simulink model "sdruFMMonoFPGA"  (R2014a)
settings: Solver=FixedStepDiscrete  SolverMode=SingleTasking  StartTime=0.0  StopTime=inf  RelTol=1e-3
PreLoadFcn:
  | monoFM = getParamsSdruFMMonoDemo;
  | tb = (atan([1, 1/2, 1/4, 1/8, 1/16, 1/32, 1/64, 1/128]));
InitFcn:
  | monoFM = getParamsSdruFMMonoDemo;
  | tb = (atan([1, 1/2, 1/4, 1/8, 1/16, 1/32, 1/64, 1/128]));
undefined symbols (not defined in the file or in its folder): mfilt
libraries: simulink x5, dspmlti4 x1, dsparch4 x1, dspsnks4 x1, sdrublksprivate x1, commsdrhw_v2 x1
CloseFcn:
  | clear monoFM;
  | clear tb
Description:
  | This model uses Universal Software Radio Peripheral (USRP) hardware with Simulink(R) to perform FM mono demodulation.
settings Model: SimulationMode=accelerator  Creator=The MathWorks Inc.
settings DataIOCC: SignalLoggingSaveFormat=ModelDataLogs  SaveOutput=off  SignalLogging=off  DSMLogging=off  SaveTime=off
settings OptimizationCC: BlockReduction=off  ConditionallyExecuteInputs=off  InlineParams=on  ExpressionDepthLimit=2147483647  SimCompilerOptimization=On
settings DebuggingCC: AlgebraicLoopMsg=error  UnderspecifiedInitializationDetection=Classic  InheritedTsInSrcMsg=none  MultiTaskCondExecSysMsg=none  IntegerOverflowMsg=none  ParameterPrecisionLossMsg=none  FcnCallInpInsideContextMsg=UseLocalSettings  StateNameClashWarn=warning
settings HardwareCC: ProdHWDeviceType=ASIC/FPGA->ASIC/FPGA  TargetBitPerLong=64  TargetBitPerPointer=64  TargetLongLongMode=on  TargetIntDivRoundTo=Zero  TargetEndianess=LittleEndian  TargetWordSize=64  TargetHWDeviceType=MATLAB Host  ProdEqTarget=off
settings SFSimCC: SFSimEnableDebug=off  SFSimOverflowDetection=off  SimIntegrity=off
settings RTWCC: CustomSourceCode=|
  | #include <stdio.h>
  | #include <stdlib.h>
settings GRTTargetCC: CombineOutputUpdateFcns=off  GRTInterface=on

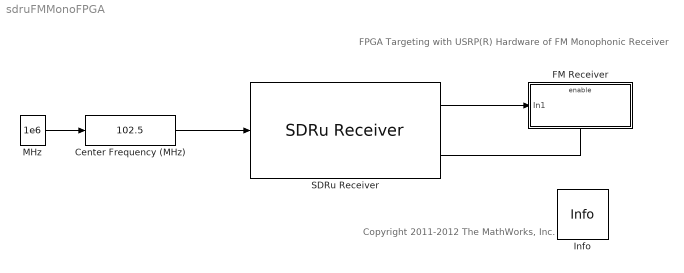
== system sdruFMMonoFPGA ==
  note: FPGA Targeting with USRP(R) Hardware of FM Monophonic Receiver
  note: Copyright 2011-2012 The MathWorks, Inc.
  Center Frequency (MHz) : simulink/Math Operations/Slider Gain  low=87.5  gain=102.5  high=108
  FM Receiver : Subsystem  TreatAsAtomicUnit=on
  Info : sdrublksprivate/Info  SystemSampleTime=-1
  MHz : Constant  Value=1e6  VectorParams1D=off  SampleTime=-1  FramePeriod=-1
  SDRu Receiver : commsdrhw_v2/SDRu Receiver  rxtx=rx  USRP2_IP='192.168.10.2'  centerFrequency=2.45e9  centerFrequencySrc=Input port  loOffset=0  loOffsetSrc=Dialog  gain=monoFM.USRPGaindB  gainSrc=Dialog  decimInterp=monoFM.USRPDecimationFactor  decimInterpSrc=Dialog  USRP2_IP_NUM=[49 57 50 46 49 54 56 46 49 48 46 50]  frameLength=monoFM.FrameLength  outputDatatype=int16  overrunUnderrunPort=off  sampleTime=1/monoFM.Fs  HOST_DATA_PORT=30000  HOST_CONTROL_PORT=30002  USRP2_DATA_PORT=32769  USRP2_CONTROL_PORT=32768  bufferMode=Guaranteed contiguous buffer  EnableBurstMode=on  NumFramesInBurst=1000
  wires:
  Center Frequency (MHz)/1 -> SDRu Receiver/1
  SDRu Receiver/2 -> FM Receiver/Enable
  MHz/1 -> Center Frequency (MHz)/1
  SDRu Receiver/1 -> FM Receiver/1(In1)

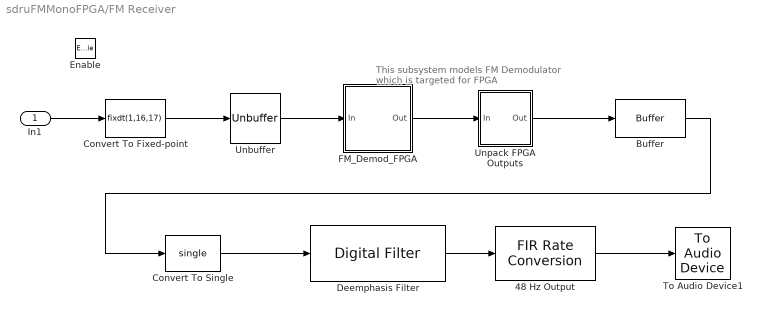
== system sdruFMMonoFPGA/FM Receiver ==
  note: This subsystem models FM Demodulator
      |  which is targeted for FPGA
  In1 : Inport
  Enable : EnablePort
  48 Hz Output : dspmlti4/FIR Rate Conversion  L=monoFM.InterpolationFactor  h=monoFM.Lowpass15k  M=monoFM.DecimationFactor  firstCoeffDataTypeStr=Inherit: Same word length as input  firstCoeffLastDataTypeStr=Inherit: Same word length as input  firstCoeffMin=[]  firstCoeffMax=[]  outputDataTypeStr=Inherit: Same as accumulator  outputLastDataTypeStr=Inherit: Same as accumulator  outputMin=[]  outputMax=[]  roundingMode=Floor  overflowMode=off  FilterSource=Specify via dialog  FilterObject=mfilt.firsrc(6,5)
  Buffer : Buffer  N=4000  TreatMby1Signals=One channel
  Convert To Fixed-point : DataTypeConversion  OutDataTypeStr=fixdt(1,16,17)  ConvertRealWorld=Stored Integer (SI)
  Convert To Single : DataTypeConversion  OutDataTypeStr=single
  Deemphasis Filter : dsparch4/Digital Filter  TypePopup=IIR (poles & zeros)  IIRFiltStruct=Direct form II transposed  AllPoleFiltStruct=Direct form  FIRFiltStruct=Direct form  CoeffSource=Specify via dialog  NumCoeffs=[1 2]  DenCoeffs=[1 0.1]  BiQuadCoeffs=[1 0.3 0.4 1 0.1 0.2]  LatticeCoeffs=[0.2 0.4]  denIgnore=on  FiltPerSampPopup=One filter per frame  IC=0  ICnum=0  ICden=0  roundingMode=Floor  overflowMode=off  ScaleValues=1  scaleValueFracLength=14  stageInFracLength=15  stageOutFracLength=15  FilterSource=dfilt object  dfiltObjectName=monoFM.DeemphasisFilter  InputProcessing=Columns as channels (frame based)
  FM_Demod_FPGA : Subsystem
  To Audio Device1 : dspsnks4/To Audio Device  deviceName=Default  inheritSampleRate=on  sampleRate=48009  deviceDatatype=Determine from input data type  autoBufferSize=on  bufferSize=4096  queueDuration=1.0  defaultOutputChannelMapping=on  outputChannelMapping=1
  Unbuffer : Unbuffer  SampleBasedProcessing=Same as frame based
  Unpack FPGA Outputs : Subsystem
  wires:
  Deemphasis Filter/1 -> 48 Hz Output/1
  48 Hz Output/1 -> To Audio Device1/1
  In1/1 -> Convert To Fixed-point/1
  Convert To Single/1 -> Deemphasis Filter/1
  Convert To Fixed-point/1 -> Unbuffer/1
  Unbuffer/1 -> FM_Demod_FPGA/1(In)
  Unpack FPGA Outputs/1(Out) -> Buffer/1
  FM_Demod_FPGA/1(Out) -> Unpack FPGA Outputs/1(In)
  Buffer/1 -> Convert To Single/1

== system sdruFMMonoFPGA/FM Receiver/FM_Demod_FPGA ==
  In : Inport
  FM Demodulator : Subsystem
  FPGA to Host : Subsystem
  Out : Outport
  wires:
  FPGA to Host/1(Out) -> Out/1
  In/1 -> FM Demodulator/1(In)
  FM Demodulator/1(Out) -> FPGA to Host/1(In)

== system sdruFMMonoFPGA/FM Receiver/Unpack FPGA Outputs ==
  note: Convert the FPGA outputs, as received from USRP(R) N210 Hardware, to FM Demodulator output format
  In : Inport
  Complex to Real-Imag : ComplexToRealImag
  Data Type Conversion2 : DataTypeConversion  OutDataTypeStr=fixdt(1,32,29)  ConvertRealWorld=Stored Integer (SI)
  Data Type Conversion4 : DataTypeConversion  OutDataTypeStr=int32  ConvertRealWorld=Stored Integer (SI)
  Data Type Conversion5 : DataTypeConversion  OutDataTypeStr=int32  ConvertRealWorld=Stored Integer (SI)
  Shift Arithmetic : ArithShift  BitShiftNumber=16  BitShiftDirection=Left
  Sum : Sum  Inputs=|++  OutDataTypeStr=int32
  Out : Outport
  wires:
  Complex to Real-Imag/2 -> Data Type Conversion5/1
  Data Type Conversion2/1 -> Out/1
  Data Type Conversion5/1 -> Sum/2
  Data Type Conversion4/1 -> Shift Arithmetic/1
  Sum/1 -> Data Type Conversion2/1
  Shift Arithmetic/1 -> Sum/1
  In/1 -> Complex to Real-Imag/1
  Complex to Real-Imag/1 -> Data Type Conversion4/1

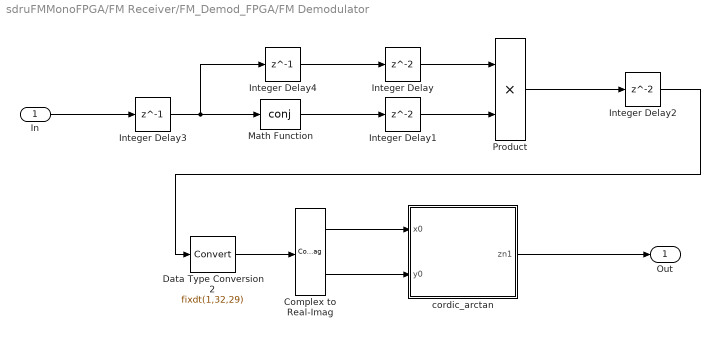
== system sdruFMMonoFPGA/FM Receiver/FM_Demod_FPGA/FM Demodulator ==
  In : Inport
  Complex to Real-Imag : ComplexToRealImag
  Data Type Conversion2 : DataTypeConversion  OutDataTypeStr=fixdt(1,32,29)
  Integer Delay : Delay
  Integer Delay1 : Delay
  Integer Delay2 : Delay
  Integer Delay3 : Delay  DelayLength=1
  Integer Delay4 : Delay  DelayLength=1
  Math Function : Math  Operator=conj  SaturateOnIntegerOverflow=on
  Product : Product  RndMeth=Zero
  cordic_arctan : Subsystem
  Out : Outport
  wires:
  Integer Delay1/1 -> Product/2
  Integer Delay/1 -> Product/1
  Integer Delay3/1 -> Integer Delay4/1, Math Function/1
  Product/1 -> Integer Delay2/1
  Complex to Real-Imag/2 -> cordic_arctan/2(y0)
  Complex to Real-Imag/1 -> cordic_arctan/1(x0)
  cordic_arctan/1(zn1) -> Out/1
  Math Function/1 -> Integer Delay1/1
  In/1 -> Integer Delay3/1
  Integer Delay4/1 -> Integer Delay/1
  Integer Delay2/1 -> Data Type Conversion2/1
  Data Type Conversion2/1 -> Complex to Real-Imag/1

== system sdruFMMonoFPGA/FM Receiver/FM_Demod_FPGA/FPGA to Host ==
  note: Convert the output of demodulator to 16 bit complex integer to match the host interface requirement of USRP(R) N210
  In : Inport
  Real-Imag to Complex : RealImagToComplex
  lsb16bits : simulink/Logic and Bit Operations/Extract Bits  bitsToExtract=Lower half  numBits=8  bitIdxRange=[0 7]  outScalingMode=Treat bit field as an integer
  msb16bits : simulink/Logic and Bit Operations/Extract Bits  bitsToExtract=Upper half  numBits=8  bitIdxRange=[0 7]  outScalingMode=Treat bit field as an integer
  Out : Outport
  wires:
  In/1 -> msb16bits/1, lsb16bits/1
  msb16bits/1 -> Real-Imag to Complex/1
  lsb16bits/1 -> Real-Imag to Complex/2
  Real-Imag to Complex/1 -> Out/1

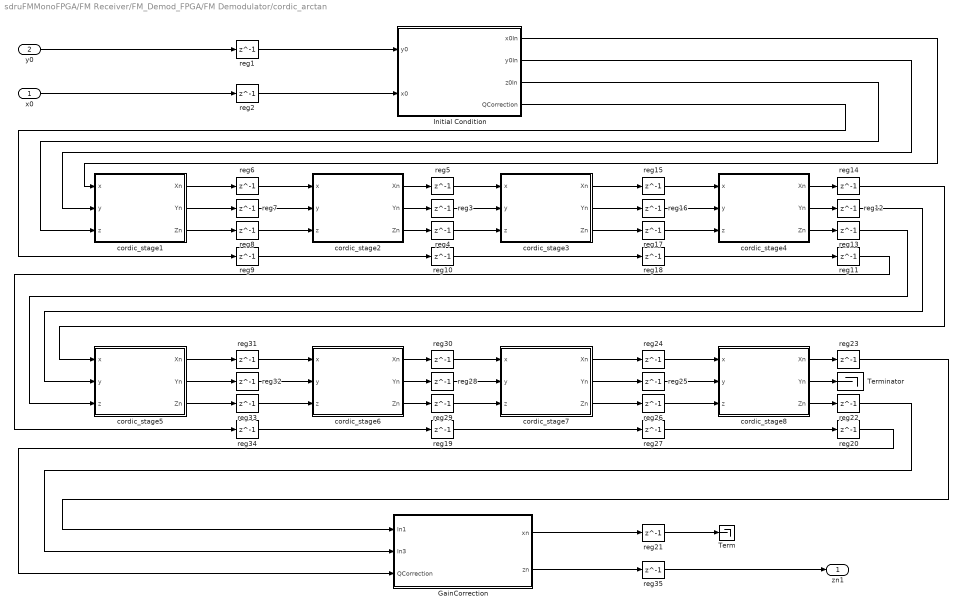
== system sdruFMMonoFPGA/FM Receiver/FM_Demod_FPGA/FM Demodulator/cordic_arctan ==
  x0 : Inport
  y0 : Inport  Port=2
  GainCorrection : Subsystem
  Initial Condition : Subsystem
  Term : Terminator
  Terminator : Terminator
  cordic_stage1 : Subsystem
  cordic_stage2 : Subsystem
  cordic_stage3 : Subsystem
  cordic_stage4 : Subsystem
  cordic_stage5 : Subsystem
  cordic_stage6 : Subsystem
  cordic_stage7 : Subsystem
  cordic_stage8 : Subsystem
  reg{1..35} (35 alike) : Delay  DelayLength=1
  zn1 : Outport
  wires:
  y0/1 -> reg1/1
  x0/1 -> reg2/1
  Initial Condition/1(x0In) -> cordic_stage1/1(x)
  Initial Condition/2(y0In) -> cordic_stage1/2(y)
  reg1/1 -> Initial Condition/1(y0)
  reg2/1 -> Initial Condition/2(x0)
  cordic_stage1/1(Xn) -> reg6/1
  cordic_stage1/2(Yn) -> reg7/1
  cordic_stage1/3(Zn) -> reg8/1
  reg6/1 -> cordic_stage2/1(x)
  reg7/1 -> cordic_stage2/2(y)
  reg8/1 -> cordic_stage2/3(z)
  cordic_stage2/1(Xn) -> reg5/1
  cordic_stage2/2(Yn) -> reg3/1
  cordic_stage2/3(Zn) -> reg4/1
  Initial Condition/3(z0In) -> cordic_stage1/3(z)
  Initial Condition/4(QCorrection) -> reg9/1
  reg9/1 -> reg10/1
  cordic_stage3/1(Xn) -> reg15/1
  cordic_stage3/2(Yn) -> reg16/1
  cordic_stage3/3(Zn) -> reg17/1
  reg15/1 -> cordic_stage4/1(x)
  reg16/1 -> cordic_stage4/2(y)
  reg17/1 -> cordic_stage4/3(z)
  cordic_stage4/1(Xn) -> reg14/1
  cordic_stage4/2(Yn) -> reg12/1
  cordic_stage4/3(Zn) -> reg13/1
  reg18/1 -> reg11/1
  reg5/1 -> cordic_stage3/1(x)
  reg3/1 -> cordic_stage3/2(y)
  reg4/1 -> cordic_stage3/3(z)
  reg10/1 -> reg18/1
  cordic_stage5/1(Xn) -> reg31/1
  cordic_stage5/2(Yn) -> reg32/1
  cordic_stage5/3(Zn) -> reg33/1
  reg31/1 -> cordic_stage6/1(x)
  reg32/1 -> cordic_stage6/2(y)
  reg33/1 -> cordic_stage6/3(z)
  cordic_stage6/1(Xn) -> reg30/1
  cordic_stage6/2(Yn) -> reg28/1
  cordic_stage6/3(Zn) -> reg29/1
  reg34/1 -> reg19/1
  cordic_stage7/1(Xn) -> reg24/1
  cordic_stage7/2(Yn) -> reg25/1
  cordic_stage7/3(Zn) -> reg26/1
  reg24/1 -> cordic_stage8/1(x)
  reg25/1 -> cordic_stage8/2(y)
  reg26/1 -> cordic_stage8/3(z)
  cordic_stage8/1(Xn) -> reg23/1
  cordic_stage8/2(Yn) -> Terminator/1
  cordic_stage8/3(Zn) -> reg22/1
  reg27/1 -> reg20/1
  reg30/1 -> cordic_stage7/1(x)
  reg28/1 -> cordic_stage7/2(y)
  reg29/1 -> cordic_stage7/3(z)
  reg19/1 -> reg27/1
  reg11/1 -> reg34/1
  reg13/1 -> cordic_stage5/3(z)
  reg12/1 -> cordic_stage5/2(y)
  reg14/1 -> cordic_stage5/1(x)
  reg20/1 -> GainCorrection/3(QCorrection)
  reg22/1 -> GainCorrection/2(In3)
  reg23/1 -> GainCorrection/1(In1)
  GainCorrection/1(xn) -> reg21/1
  GainCorrection/2(zn) -> reg35/1
  reg35/1 -> zn1/1
  reg21/1 -> Term/1

== system sdruFMMonoFPGA/FM Receiver/FM_Demod_FPGA/FM Demodulator/cordic_arctan/GainCorrection ==
  In1 : Inport
  In3 : Inport  Port=2
  QCorrection : Inport  Port=3
  AngleCorrection : Subsystem
  Gain : Gain  Gain=1/sqrt(2*(1+2^-2)*(1+2^-4)*(1+2^-6)*(1+2^-8)*(1+2^-10)*(1+2^-12)*(1+2^-14))  OutDataTypeStr=Inherit: Same as input
  xn : Outport
  zn : Outport  Port=2
  wires:
  QCorrection/1 -> AngleCorrection/1(In2)
  AngleCorrection/1(Out1) -> zn/1
  Gain/1 -> xn/1
  In3/1 -> AngleCorrection/2(In1)
  In1/1 -> Gain/1

== system sdruFMMonoFPGA/FM Receiver/FM_Demod_FPGA/FM Demodulator/cordic_arctan/Initial Condition ==
  y0 : Inport
  x0 : Inport  Port=2
  Subsystem : Subsystem
  Subsystem1 : Subsystem
  Subsystem2 : Subsystem
  zInitial : Constant  Value=0  OutDataTypeStr=fixdt(1,32,29)  SampleTime=-1
  x0In : Outport
  y0In : Outport  Port=2
  z0In : Outport  Port=3
  QCorrection : Outport  Port=4
  wires:
  Subsystem2/1(Quadrant) -> QCorrection/1
  Subsystem1/2(negative) -> Subsystem2/1(In1)
  Subsystem/1(negative) -> Subsystem2/2(In2)
  Subsystem1/1(magnitude) -> x0In/1
  x0/1 -> Subsystem1/1(In1)
  Subsystem/2(magnitude) -> y0In/1
  zInitial/1 -> z0In/1
  y0/1 -> Subsystem/1(In1)

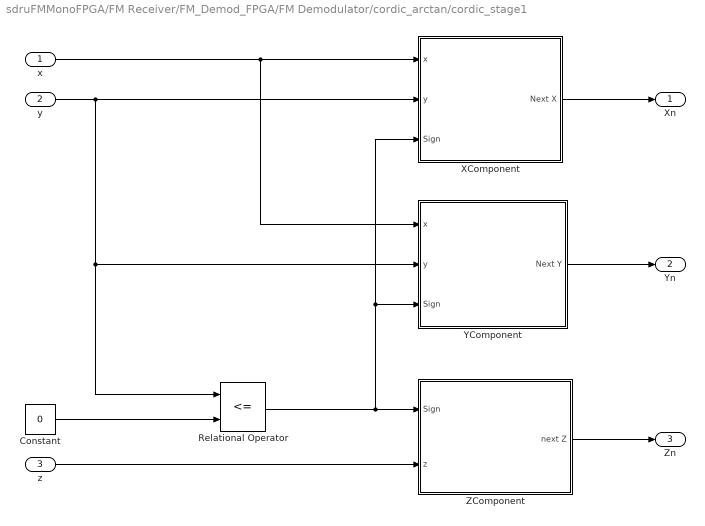
== system sdruFMMonoFPGA/FM Receiver/FM_Demod_FPGA/FM Demodulator/cordic_arctan/cordic_stage1 ==
  x : Inport
  y : Inport  Port=2
  z : Inport  Port=3
  Constant : Constant  Value=0  OutDataTypeStr=Inherit: Inherit via back propagation
  Relational Operator : RelationalOperator  Operator=<=  OutDataTypeStr=boolean  InputSameDT=on
  XComponent : Subsystem
  YComponent : Subsystem
  ZComponent : Subsystem
  Xn : Outport
  Yn : Outport  Port=2
  Zn : Outport  Port=3
  wires:
  Constant/1 -> Relational Operator/2
  ZComponent/1(next Z) -> Zn/1
  z/1 -> ZComponent/2(z)
  YComponent/1(Next Y) -> Yn/1
  XComponent/1(Next X) -> Xn/1
  x/1 -> YComponent/1(x), XComponent/1(x)
  Relational Operator/1 -> ZComponent/1(Sign), YComponent/3(Sign), XComponent/3(Sign)
  y/1 -> XComponent/2(y), Relational Operator/1, YComponent/2(y)

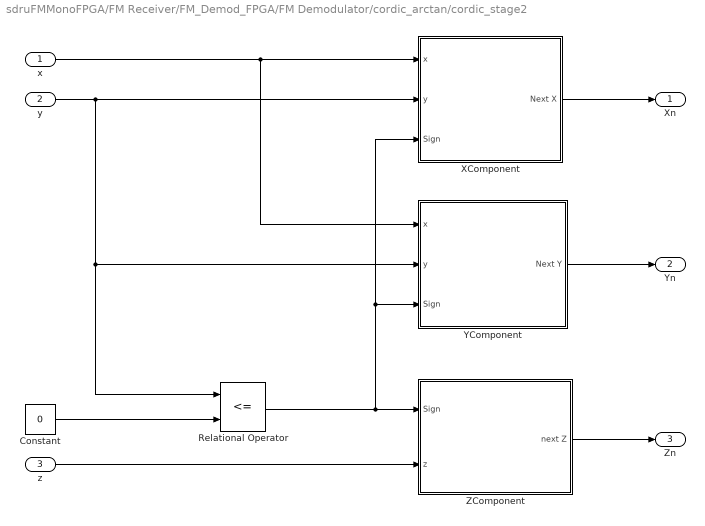
== system sdruFMMonoFPGA/FM Receiver/FM_Demod_FPGA/FM Demodulator/cordic_arctan/cordic_stage2 ==
  x : Inport
  y : Inport  Port=2
  z : Inport  Port=3
  Constant : Constant  Value=0  OutDataTypeStr=Inherit: Inherit via back propagation
  Relational Operator : RelationalOperator  Operator=<=  OutDataTypeStr=boolean  InputSameDT=on
  XComponent : Subsystem
  YComponent : Subsystem
  ZComponent : Subsystem
  Xn : Outport
  Yn : Outport  Port=2
  Zn : Outport  Port=3
  wires:
  y/1 -> YComponent/2(y), Relational Operator/1, XComponent/2(y)
  Relational Operator/1 -> XComponent/3(Sign), YComponent/3(Sign), ZComponent/1(Sign)
  x/1 -> XComponent/1(x), YComponent/1(x)
  XComponent/1(Next X) -> Xn/1
  YComponent/1(Next Y) -> Yn/1
  z/1 -> ZComponent/2(z)
  ZComponent/1(next Z) -> Zn/1
  Constant/1 -> Relational Operator/2

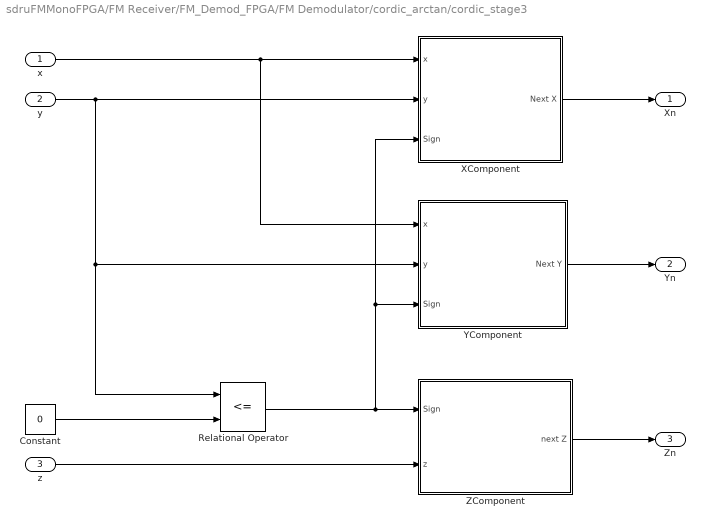
== system sdruFMMonoFPGA/FM Receiver/FM_Demod_FPGA/FM Demodulator/cordic_arctan/cordic_stage3 ==
  x : Inport
  y : Inport  Port=2
  z : Inport  Port=3
  Constant : Constant  Value=0  OutDataTypeStr=Inherit: Inherit via back propagation
  Relational Operator : RelationalOperator  Operator=<=  OutDataTypeStr=boolean  InputSameDT=on
  XComponent : Subsystem
  YComponent : Subsystem
  ZComponent : Subsystem
  Xn : Outport
  Yn : Outport  Port=2
  Zn : Outport  Port=3
  wires:
  Constant/1 -> Relational Operator/2
  ZComponent/1(next Z) -> Zn/1
  z/1 -> ZComponent/2(z)
  YComponent/1(Next Y) -> Yn/1
  XComponent/1(Next X) -> Xn/1
  x/1 -> YComponent/1(x), XComponent/1(x)
  Relational Operator/1 -> ZComponent/1(Sign), YComponent/3(Sign), XComponent/3(Sign)
  y/1 -> XComponent/2(y), Relational Operator/1, YComponent/2(y)

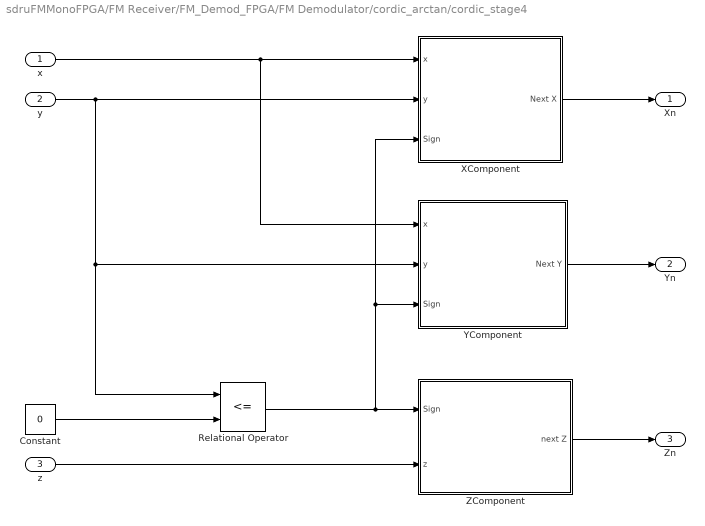
== system sdruFMMonoFPGA/FM Receiver/FM_Demod_FPGA/FM Demodulator/cordic_arctan/cordic_stage4 ==
  x : Inport
  y : Inport  Port=2
  z : Inport  Port=3
  Constant : Constant  Value=0  OutDataTypeStr=Inherit: Inherit via back propagation
  Relational Operator : RelationalOperator  Operator=<=  OutDataTypeStr=boolean  InputSameDT=on
  XComponent : Subsystem
  YComponent : Subsystem
  ZComponent : Subsystem
  Xn : Outport
  Yn : Outport  Port=2
  Zn : Outport  Port=3
  wires:
  y/1 -> YComponent/2(y), Relational Operator/1, XComponent/2(y)
  Relational Operator/1 -> XComponent/3(Sign), YComponent/3(Sign), ZComponent/1(Sign)
  x/1 -> XComponent/1(x), YComponent/1(x)
  XComponent/1(Next X) -> Xn/1
  YComponent/1(Next Y) -> Yn/1
  z/1 -> ZComponent/2(z)
  ZComponent/1(next Z) -> Zn/1
  Constant/1 -> Relational Operator/2

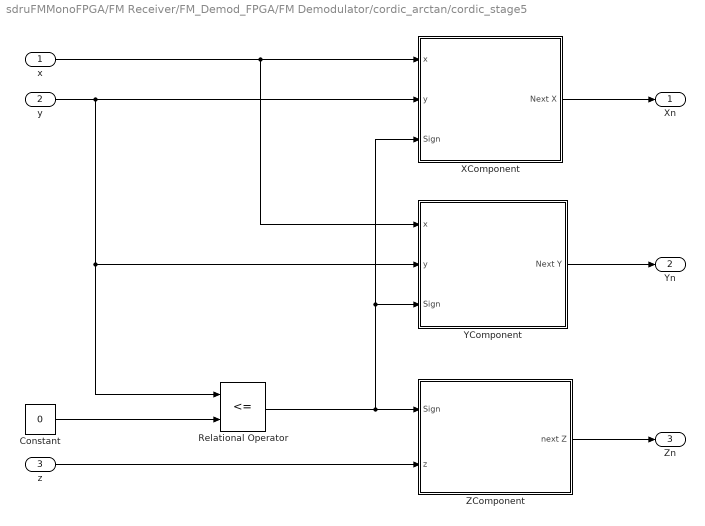
== system sdruFMMonoFPGA/FM Receiver/FM_Demod_FPGA/FM Demodulator/cordic_arctan/cordic_stage5 ==
  x : Inport
  y : Inport  Port=2
  z : Inport  Port=3
  Constant : Constant  Value=0  OutDataTypeStr=Inherit: Inherit via back propagation
  Relational Operator : RelationalOperator  Operator=<=  OutDataTypeStr=boolean  InputSameDT=on
  XComponent : Subsystem
  YComponent : Subsystem
  ZComponent : Subsystem
  Xn : Outport
  Yn : Outport  Port=2
  Zn : Outport  Port=3
  wires:
  Constant/1 -> Relational Operator/2
  ZComponent/1(next Z) -> Zn/1
  z/1 -> ZComponent/2(z)
  YComponent/1(Next Y) -> Yn/1
  XComponent/1(Next X) -> Xn/1
  x/1 -> YComponent/1(x), XComponent/1(x)
  Relational Operator/1 -> ZComponent/1(Sign), YComponent/3(Sign), XComponent/3(Sign)
  y/1 -> XComponent/2(y), Relational Operator/1, YComponent/2(y)

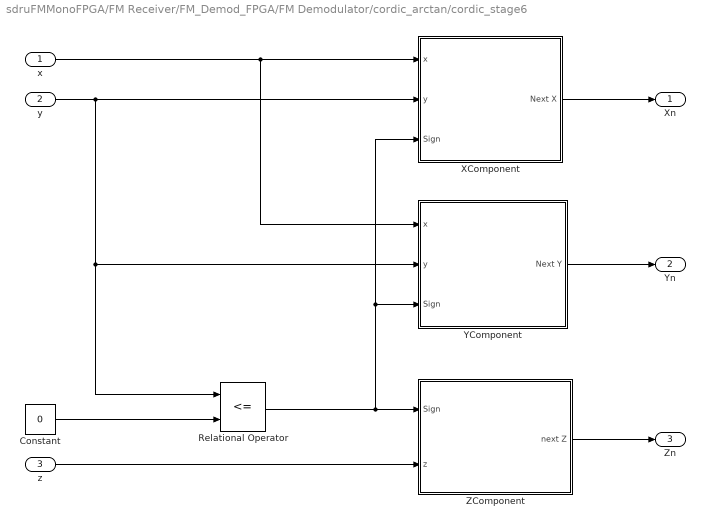
== system sdruFMMonoFPGA/FM Receiver/FM_Demod_FPGA/FM Demodulator/cordic_arctan/cordic_stage6 ==
  x : Inport
  y : Inport  Port=2
  z : Inport  Port=3
  Constant : Constant  Value=0  OutDataTypeStr=Inherit: Inherit via back propagation
  Relational Operator : RelationalOperator  Operator=<=  OutDataTypeStr=boolean  InputSameDT=on
  XComponent : Subsystem
  YComponent : Subsystem
  ZComponent : Subsystem
  Xn : Outport
  Yn : Outport  Port=2
  Zn : Outport  Port=3
  wires:
  y/1 -> YComponent/2(y), Relational Operator/1, XComponent/2(y)
  Relational Operator/1 -> XComponent/3(Sign), YComponent/3(Sign), ZComponent/1(Sign)
  x/1 -> XComponent/1(x), YComponent/1(x)
  XComponent/1(Next X) -> Xn/1
  YComponent/1(Next Y) -> Yn/1
  z/1 -> ZComponent/2(z)
  ZComponent/1(next Z) -> Zn/1
  Constant/1 -> Relational Operator/2

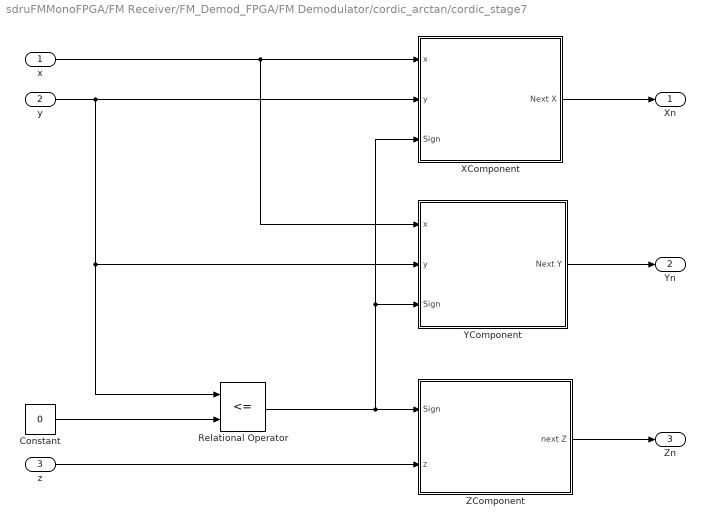
== system sdruFMMonoFPGA/FM Receiver/FM_Demod_FPGA/FM Demodulator/cordic_arctan/cordic_stage7 ==
  x : Inport
  y : Inport  Port=2
  z : Inport  Port=3
  Constant : Constant  Value=0  OutDataTypeStr=Inherit: Inherit via back propagation
  Relational Operator : RelationalOperator  Operator=<=  OutDataTypeStr=boolean  InputSameDT=on
  XComponent : Subsystem
  YComponent : Subsystem
  ZComponent : Subsystem
  Xn : Outport
  Yn : Outport  Port=2
  Zn : Outport  Port=3
  wires:
  Constant/1 -> Relational Operator/2
  ZComponent/1(next Z) -> Zn/1
  z/1 -> ZComponent/2(z)
  YComponent/1(Next Y) -> Yn/1
  XComponent/1(Next X) -> Xn/1
  x/1 -> YComponent/1(x), XComponent/1(x)
  Relational Operator/1 -> ZComponent/1(Sign), YComponent/3(Sign), XComponent/3(Sign)
  y/1 -> XComponent/2(y), Relational Operator/1, YComponent/2(y)

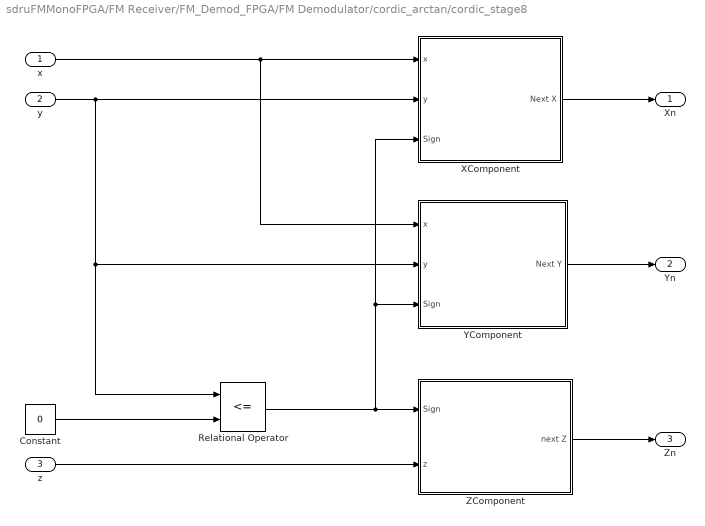
== system sdruFMMonoFPGA/FM Receiver/FM_Demod_FPGA/FM Demodulator/cordic_arctan/cordic_stage8 ==
  x : Inport
  y : Inport  Port=2
  z : Inport  Port=3
  Constant : Constant  Value=0  OutDataTypeStr=Inherit: Inherit via back propagation
  Relational Operator : RelationalOperator  Operator=<=  OutDataTypeStr=boolean  InputSameDT=on
  XComponent : Subsystem
  YComponent : Subsystem
  ZComponent : Subsystem
  Xn : Outport
  Yn : Outport  Port=2
  Zn : Outport  Port=3
  wires:
  y/1 -> YComponent/2(y), Relational Operator/1, XComponent/2(y)
  Relational Operator/1 -> XComponent/3(Sign), YComponent/3(Sign), ZComponent/1(Sign)
  x/1 -> XComponent/1(x), YComponent/1(x)
  XComponent/1(Next X) -> Xn/1
  YComponent/1(Next Y) -> Yn/1
  z/1 -> ZComponent/2(z)
  ZComponent/1(next Z) -> Zn/1
  Constant/1 -> Relational Operator/2

== system sdruFMMonoFPGA/FM Receiver/FM_Demod_FPGA/FM Demodulator/cordic_arctan/GainCorrection/AngleCorrection ==
  In2 : Inport
  In1 : Inport  Port=2
  Constant1 : Constant  Value=pi  OutDataTypeStr=fixdt(1,16,13)  SampleTime=-1
  Gain1 : Gain  Gain=-1  OutDataTypeStr=Inherit: Inherit via back propagation
  Gain2 : Gain  Gain=-1  OutDataTypeStr=Inherit: Inherit via back propagation
  Multiport Switch : MultiPortSwitch  DataPortOrder=Zero-based contiguous  Inputs=4  zeroidx=on
  Sum : Sum  Inputs=|-+  OutDataTypeStr=Inherit: Same as first input
  Sum1 : Sum  Inputs=|++  OutDataTypeStr=Inherit: Same as first input
  Out1 : Outport
  wires:
  Sum1/1 -> Multiport Switch/5
  Gain1/1 -> Sum1/2
  Multiport Switch/1 -> Out1/1
  Constant1/1 -> Gain1/1, Sum/2
  Sum/1 -> Multiport Switch/3
  Gain2/1 -> Multiport Switch/4
  In1/1 -> Sum1/1, Gain2/1, Sum/1, Multiport Switch/2
  In2/1 -> Multiport Switch/1

== system sdruFMMonoFPGA/FM Receiver/FM_Demod_FPGA/FM Demodulator/cordic_arctan/Initial Condition/Subsystem ==
  In1 : Inport
  Compare To Zero : simulink/Logic and Bit Operations/Compare To Zero  relop=<  OutDataTypeStr=uint8  ZeroCross=off
  Gain : Gain  Gain=-1  OutDataTypeStr=Inherit: Same as input
  Switch : Switch  Threshold=1
  negative : Outport
  magnitude : Outport  Port=2
  wires:
  Switch/1 -> magnitude/1
  Gain/1 -> Switch/1
  Compare To Zero/1 -> Switch/2, negative/1
  In1/1 -> Switch/3, Gain/1, Compare To Zero/1

== system sdruFMMonoFPGA/FM Receiver/FM_Demod_FPGA/FM Demodulator/cordic_arctan/Initial Condition/Subsystem1 ==
  In1 : Inport
  Compare To Zero : simulink/Logic and Bit Operations/Compare To Zero  relop=<  OutDataTypeStr=uint8  ZeroCross=off
  Gain : Gain  Gain=-1  OutDataTypeStr=Inherit: Same as input
  Switch : Switch  Threshold=1
  magnitude : Outport
  negative : Outport  Port=2
  wires:
  In1/1 -> Compare To Zero/1, Gain/1, Switch/3
  Compare To Zero/1 -> Switch/2, negative/1
  Gain/1 -> Switch/1
  Switch/1 -> magnitude/1

== system sdruFMMonoFPGA/FM Receiver/FM_Demod_FPGA/FM Demodulator/cordic_arctan/Initial Condition/Subsystem2 ==
  In1 : Inport
  In2 : Inport  Port=2
  Gain : Gain  Gain=2  OutDataTypeStr=Inherit: Same as input
  Sum : Sum  Inputs=|++
  Quadrant : Outport
  wires:
  Sum/1 -> Quadrant/1
  In1/1 -> Sum/1
  Gain/1 -> Sum/2
  In2/1 -> Gain/1

== system sdruFMMonoFPGA/FM Receiver/FM_Demod_FPGA/FM Demodulator/cordic_arctan/cordic_stage1/XComponent ==
  x : Inport
  y : Inport  Port=2
  Sign : Inport  Port=3
  Logical Not : Logic  Operator=NOT  AllPortsSameDT=off  OutDataTypeStr=boolean
  ShiftArith : ArithShift
  ZAccumulator2 : Subsystem
  Next X : Outport
  wires:
  Sign/1 -> Logical Not/1
  y/1 -> ShiftArith/1
  ZAccumulator2/1(Out1) -> Next X/1
  ShiftArith/1 -> ZAccumulator2/1(y)
  Logical Not/1 -> ZAccumulator2/2(op)
  x/1 -> ZAccumulator2/3(x)

== system sdruFMMonoFPGA/FM Receiver/FM_Demod_FPGA/FM Demodulator/cordic_arctan/cordic_stage1/YComponent ==
  x : Inport
  y : Inport  Port=2
  Sign : Inport  Port=3
  Shift Arith : ArithShift
  ZAccumulator2 : Subsystem
  Next Y : Outport
  wires:
  ZAccumulator2/1(Out1) -> Next Y/1
  x/1 -> Shift Arith/1
  Shift Arith/1 -> ZAccumulator2/1(x)
  Sign/1 -> ZAccumulator2/2(op)
  y/1 -> ZAccumulator2/3(y)

== system sdruFMMonoFPGA/FM Receiver/FM_Demod_FPGA/FM Demodulator/cordic_arctan/cordic_stage1/ZComponent ==
  Sign : Inport
  z : Inport  Port=2
  Constant : Constant  Value=tb(1)  OutDataTypeStr=fixdt(1,16,15)
  Logical Not : Logic  Operator=NOT  AllPortsSameDT=off  OutDataTypeStr=boolean
  ZAccumulator2 : Subsystem
  next Z : Outport
  wires:
  Constant/1 -> ZAccumulator2/3(y)
  Logical Not/1 -> ZAccumulator2/1(op)
  Sign/1 -> Logical Not/1
  z/1 -> ZAccumulator2/2(x)
  ZAccumulator2/1(Out1) -> next Z/1

== system sdruFMMonoFPGA/FM Receiver/FM_Demod_FPGA/FM Demodulator/cordic_arctan/cordic_stage2/XComponent ==
  x : Inport
  y : Inport  Port=2
  Sign : Inport  Port=3
  Logical Not : Logic  Operator=NOT  AllPortsSameDT=off  OutDataTypeStr=boolean
  ShiftArith : ArithShift
  ZAccumulator2 : Subsystem
  Next X : Outport
  wires:
  x/1 -> ZAccumulator2/3(x)
  Logical Not/1 -> ZAccumulator2/2(op)
  ShiftArith/1 -> ZAccumulator2/1(y)
  ZAccumulator2/1(Out1) -> Next X/1
  y/1 -> ShiftArith/1
  Sign/1 -> Logical Not/1

== system sdruFMMonoFPGA/FM Receiver/FM_Demod_FPGA/FM Demodulator/cordic_arctan/cordic_stage2/YComponent ==
  x : Inport
  y : Inport  Port=2
  Sign : Inport  Port=3
  Shift Arith : ArithShift
  ZAccumulator2 : Subsystem
  Next Y : Outport
  wires:
  y/1 -> ZAccumulator2/3(y)
  Sign/1 -> ZAccumulator2/2(op)
  Shift Arith/1 -> ZAccumulator2/1(x)
  x/1 -> Shift Arith/1
  ZAccumulator2/1(Out1) -> Next Y/1

== system sdruFMMonoFPGA/FM Receiver/FM_Demod_FPGA/FM Demodulator/cordic_arctan/cordic_stage2/ZComponent ==
  Sign : Inport
  z : Inport  Port=2
  Constant : Constant  Value=tb(2)  OutDataTypeStr=fixdt(1,16,15)
  Logical Not : Logic  Operator=NOT  AllPortsSameDT=off  OutDataTypeStr=boolean
  ZAccumulator2 : Subsystem
  next Z : Outport
  wires:
  ZAccumulator2/1(Out1) -> next Z/1
  z/1 -> ZAccumulator2/2(x)
  Sign/1 -> Logical Not/1
  Logical Not/1 -> ZAccumulator2/1(op)
  Constant/1 -> ZAccumulator2/3(y)

== system sdruFMMonoFPGA/FM Receiver/FM_Demod_FPGA/FM Demodulator/cordic_arctan/cordic_stage3/XComponent ==
  x : Inport
  y : Inport  Port=2
  Sign : Inport  Port=3
  Logical Not : Logic  Operator=NOT  AllPortsSameDT=off  OutDataTypeStr=boolean
  ShiftArith : ArithShift
  ZAccumulator2 : Subsystem
  Next X : Outport
  wires:
  Sign/1 -> Logical Not/1
  y/1 -> ShiftArith/1
  ZAccumulator2/1(Out1) -> Next X/1
  ShiftArith/1 -> ZAccumulator2/1(y)
  Logical Not/1 -> ZAccumulator2/2(op)
  x/1 -> ZAccumulator2/3(x)

== system sdruFMMonoFPGA/FM Receiver/FM_Demod_FPGA/FM Demodulator/cordic_arctan/cordic_stage3/YComponent ==
  x : Inport
  y : Inport  Port=2
  Sign : Inport  Port=3
  Shift Arith : ArithShift
  ZAccumulator2 : Subsystem
  Next Y : Outport
  wires:
  ZAccumulator2/1(Out1) -> Next Y/1
  x/1 -> Shift Arith/1
  Shift Arith/1 -> ZAccumulator2/1(x)
  Sign/1 -> ZAccumulator2/2(op)
  y/1 -> ZAccumulator2/3(y)

== system sdruFMMonoFPGA/FM Receiver/FM_Demod_FPGA/FM Demodulator/cordic_arctan/cordic_stage3/ZComponent ==
  Sign : Inport
  z : Inport  Port=2
  Constant : Constant  Value=tb(3)  OutDataTypeStr=fixdt(1,16,15)
  Logical Not : Logic  Operator=NOT  AllPortsSameDT=off  OutDataTypeStr=boolean
  ZAccumulator2 : Subsystem
  next Z : Outport
  wires:
  Constant/1 -> ZAccumulator2/3(y)
  Logical Not/1 -> ZAccumulator2/1(op)
  Sign/1 -> Logical Not/1
  z/1 -> ZAccumulator2/2(x)
  ZAccumulator2/1(Out1) -> next Z/1

== system sdruFMMonoFPGA/FM Receiver/FM_Demod_FPGA/FM Demodulator/cordic_arctan/cordic_stage4/XComponent ==
  x : Inport
  y : Inport  Port=2
  Sign : Inport  Port=3
  Logical Not : Logic  Operator=NOT  AllPortsSameDT=off  OutDataTypeStr=boolean
  ShiftArith : ArithShift
  ZAccumulator2 : Subsystem
  Next X : Outport
  wires:
  x/1 -> ZAccumulator2/3(x)
  Logical Not/1 -> ZAccumulator2/2(op)
  ShiftArith/1 -> ZAccumulator2/1(y)
  ZAccumulator2/1(Out1) -> Next X/1
  y/1 -> ShiftArith/1
  Sign/1 -> Logical Not/1

== system sdruFMMonoFPGA/FM Receiver/FM_Demod_FPGA/FM Demodulator/cordic_arctan/cordic_stage4/YComponent ==
  x : Inport
  y : Inport  Port=2
  Sign : Inport  Port=3
  Shift Arith : ArithShift
  ZAccumulator2 : Subsystem
  Next Y : Outport
  wires:
  y/1 -> ZAccumulator2/3(y)
  Sign/1 -> ZAccumulator2/2(op)
  Shift Arith/1 -> ZAccumulator2/1(x)
  x/1 -> Shift Arith/1
  ZAccumulator2/1(Out1) -> Next Y/1

== system sdruFMMonoFPGA/FM Receiver/FM_Demod_FPGA/FM Demodulator/cordic_arctan/cordic_stage4/ZComponent ==
  Sign : Inport
  z : Inport  Port=2
  Constant : Constant  Value=tb(4)  OutDataTypeStr=fixdt(1,16,15)
  Logical Not : Logic  Operator=NOT  AllPortsSameDT=off  OutDataTypeStr=boolean
  ZAccumulator2 : Subsystem
  next Z : Outport
  wires:
  ZAccumulator2/1(Out1) -> next Z/1
  z/1 -> ZAccumulator2/2(x)
  Sign/1 -> Logical Not/1
  Logical Not/1 -> ZAccumulator2/1(op)
  Constant/1 -> ZAccumulator2/3(y)

== system sdruFMMonoFPGA/FM Receiver/FM_Demod_FPGA/FM Demodulator/cordic_arctan/cordic_stage5/XComponent ==
  x : Inport
  y : Inport  Port=2
  Sign : Inport  Port=3
  Logical Not : Logic  Operator=NOT  AllPortsSameDT=off  OutDataTypeStr=boolean
  ShiftArith : ArithShift
  ZAccumulator2 : Subsystem
  Next X : Outport
  wires:
  Sign/1 -> Logical Not/1
  y/1 -> ShiftArith/1
  ZAccumulator2/1(Out1) -> Next X/1
  ShiftArith/1 -> ZAccumulator2/1(y)
  Logical Not/1 -> ZAccumulator2/2(op)
  x/1 -> ZAccumulator2/3(x)

== system sdruFMMonoFPGA/FM Receiver/FM_Demod_FPGA/FM Demodulator/cordic_arctan/cordic_stage5/YComponent ==
  x : Inport
  y : Inport  Port=2
  Sign : Inport  Port=3
  Shift Arith : ArithShift
  ZAccumulator2 : Subsystem
  Next Y : Outport
  wires:
  ZAccumulator2/1(Out1) -> Next Y/1
  x/1 -> Shift Arith/1
  Shift Arith/1 -> ZAccumulator2/1(x)
  Sign/1 -> ZAccumulator2/2(op)
  y/1 -> ZAccumulator2/3(y)

== system sdruFMMonoFPGA/FM Receiver/FM_Demod_FPGA/FM Demodulator/cordic_arctan/cordic_stage5/ZComponent ==
  Sign : Inport
  z : Inport  Port=2
  Constant : Constant  Value=tb(5)  OutDataTypeStr=fixdt(1,16,15)
  Logical Not : Logic  Operator=NOT  AllPortsSameDT=off  OutDataTypeStr=boolean
  ZAccumulator2 : Subsystem
  next Z : Outport
  wires:
  Constant/1 -> ZAccumulator2/3(y)
  Logical Not/1 -> ZAccumulator2/1(op)
  Sign/1 -> Logical Not/1
  z/1 -> ZAccumulator2/2(x)
  ZAccumulator2/1(Out1) -> next Z/1

== system sdruFMMonoFPGA/FM Receiver/FM_Demod_FPGA/FM Demodulator/cordic_arctan/cordic_stage6/XComponent ==
  x : Inport
  y : Inport  Port=2
  Sign : Inport  Port=3
  Logical Not : Logic  Operator=NOT  AllPortsSameDT=off  OutDataTypeStr=boolean
  ShiftArith : ArithShift
  ZAccumulator2 : Subsystem
  Next X : Outport
  wires:
  x/1 -> ZAccumulator2/3(x)
  Logical Not/1 -> ZAccumulator2/2(op)
  ShiftArith/1 -> ZAccumulator2/1(y)
  ZAccumulator2/1(Out1) -> Next X/1
  y/1 -> ShiftArith/1
  Sign/1 -> Logical Not/1

== system sdruFMMonoFPGA/FM Receiver/FM_Demod_FPGA/FM Demodulator/cordic_arctan/cordic_stage6/YComponent ==
  x : Inport
  y : Inport  Port=2
  Sign : Inport  Port=3
  Shift Arith : ArithShift
  ZAccumulator2 : Subsystem
  Next Y : Outport
  wires:
  y/1 -> ZAccumulator2/3(y)
  Sign/1 -> ZAccumulator2/2(op)
  Shift Arith/1 -> ZAccumulator2/1(x)
  x/1 -> Shift Arith/1
  ZAccumulator2/1(Out1) -> Next Y/1

== system sdruFMMonoFPGA/FM Receiver/FM_Demod_FPGA/FM Demodulator/cordic_arctan/cordic_stage6/ZComponent ==
  Sign : Inport
  z : Inport  Port=2
  Constant : Constant  Value=tb(6)  OutDataTypeStr=fixdt(1,16,15)
  Logical Not : Logic  Operator=NOT  AllPortsSameDT=off  OutDataTypeStr=boolean
  ZAccumulator2 : Subsystem
  next Z : Outport
  wires:
  ZAccumulator2/1(Out1) -> next Z/1
  z/1 -> ZAccumulator2/2(x)
  Sign/1 -> Logical Not/1
  Logical Not/1 -> ZAccumulator2/1(op)
  Constant/1 -> ZAccumulator2/3(y)

== system sdruFMMonoFPGA/FM Receiver/FM_Demod_FPGA/FM Demodulator/cordic_arctan/cordic_stage7/XComponent ==
  x : Inport
  y : Inport  Port=2
  Sign : Inport  Port=3
  Logical Not : Logic  Operator=NOT  AllPortsSameDT=off  OutDataTypeStr=boolean
  ShiftArith : ArithShift
  ZAccumulator2 : Subsystem
  Next X : Outport
  wires:
  Sign/1 -> Logical Not/1
  y/1 -> ShiftArith/1
  ZAccumulator2/1(Out1) -> Next X/1
  ShiftArith/1 -> ZAccumulator2/1(y)
  Logical Not/1 -> ZAccumulator2/2(op)
  x/1 -> ZAccumulator2/3(x)

== system sdruFMMonoFPGA/FM Receiver/FM_Demod_FPGA/FM Demodulator/cordic_arctan/cordic_stage7/YComponent ==
  x : Inport
  y : Inport  Port=2
  Sign : Inport  Port=3
  Shift Arith : ArithShift
  ZAccumulator2 : Subsystem
  Next Y : Outport
  wires:
  ZAccumulator2/1(Out1) -> Next Y/1
  x/1 -> Shift Arith/1
  Shift Arith/1 -> ZAccumulator2/1(x)
  Sign/1 -> ZAccumulator2/2(op)
  y/1 -> ZAccumulator2/3(y)

== system sdruFMMonoFPGA/FM Receiver/FM_Demod_FPGA/FM Demodulator/cordic_arctan/cordic_stage7/ZComponent ==
  Sign : Inport
  z : Inport  Port=2
  Constant : Constant  Value=tb(7)  OutDataTypeStr=fixdt(1,16,15)
  Logical Not : Logic  Operator=NOT  AllPortsSameDT=off  OutDataTypeStr=boolean
  ZAccumulator2 : Subsystem
  next Z : Outport
  wires:
  Constant/1 -> ZAccumulator2/3(y)
  Logical Not/1 -> ZAccumulator2/1(op)
  Sign/1 -> Logical Not/1
  z/1 -> ZAccumulator2/2(x)
  ZAccumulator2/1(Out1) -> next Z/1

== system sdruFMMonoFPGA/FM Receiver/FM_Demod_FPGA/FM Demodulator/cordic_arctan/cordic_stage8/XComponent ==
  x : Inport
  y : Inport  Port=2
  Sign : Inport  Port=3
  Logical Not : Logic  Operator=NOT  AllPortsSameDT=off  OutDataTypeStr=boolean
  ShiftArith : ArithShift
  ZAccumulator2 : Subsystem
  Next X : Outport
  wires:
  x/1 -> ZAccumulator2/3(x)
  Logical Not/1 -> ZAccumulator2/2(op)
  ShiftArith/1 -> ZAccumulator2/1(y)
  ZAccumulator2/1(Out1) -> Next X/1
  y/1 -> ShiftArith/1
  Sign/1 -> Logical Not/1

== system sdruFMMonoFPGA/FM Receiver/FM_Demod_FPGA/FM Demodulator/cordic_arctan/cordic_stage8/YComponent ==
  x : Inport
  y : Inport  Port=2
  Sign : Inport  Port=3
  Shift Arith : ArithShift
  ZAccumulator2 : Subsystem
  Next Y : Outport
  wires:
  y/1 -> ZAccumulator2/3(y)
  Sign/1 -> ZAccumulator2/2(op)
  Shift Arith/1 -> ZAccumulator2/1(x)
  x/1 -> Shift Arith/1
  ZAccumulator2/1(Out1) -> Next Y/1

== system sdruFMMonoFPGA/FM Receiver/FM_Demod_FPGA/FM Demodulator/cordic_arctan/cordic_stage8/ZComponent ==
  Sign : Inport
  z : Inport  Port=2
  Constant : Constant  Value=tb(8)  OutDataTypeStr=fixdt(1,16,15)
  Logical Not : Logic  Operator=NOT  AllPortsSameDT=off  OutDataTypeStr=boolean
  ZAccumulator2 : Subsystem
  next Z : Outport
  wires:
  ZAccumulator2/1(Out1) -> next Z/1
  z/1 -> ZAccumulator2/2(x)
  Sign/1 -> Logical Not/1
  Logical Not/1 -> ZAccumulator2/1(op)
  Constant/1 -> ZAccumulator2/3(y)

== system sdruFMMonoFPGA/FM Receiver/FM_Demod_FPGA/FM Demodulator/cordic_arctan/cordic_stage1/XComponent/ZAccumulator2 ==
  y : Inport
  op : Inport  Port=2
  x : Inport  Port=3
  Sum1 : Sum  Inputs=|++  OutDataTypeStr=Inherit: Same as first input
  Sum2 : Sum  Inputs=|+-  OutDataTypeStr=Inherit: Same as first input
  Switch : Switch  Criteria=u2 ~= 0
  Out1 : Outport
  wires:
  Switch/1 -> Out1/1
  Sum1/1 -> Switch/1
  op/1 -> Switch/2
  Sum2/1 -> Switch/3
  x/1 -> Sum1/1, Sum2/1
  y/1 -> Sum1/2, Sum2/2

== system sdruFMMonoFPGA/FM Receiver/FM_Demod_FPGA/FM Demodulator/cordic_arctan/cordic_stage1/YComponent/ZAccumulator2 ==
  x : Inport
  op : Inport  Port=2
  y : Inport  Port=3
  Sum1 : Sum  Inputs=|++  OutDataTypeStr=Inherit: Same as first input
  Sum2 : Sum  Inputs=|+-  OutDataTypeStr=Inherit: Same as first input
  Switch : Switch  Criteria=u2 ~= 0  InputSameDT=on
  Out1 : Outport
  wires:
  x/1 -> Sum1/2, Sum2/2
  Switch/1 -> Out1/1
  Sum1/1 -> Switch/1
  op/1 -> Switch/2
  Sum2/1 -> Switch/3
  y/1 -> Sum1/1, Sum2/1

== system sdruFMMonoFPGA/FM Receiver/FM_Demod_FPGA/FM Demodulator/cordic_arctan/cordic_stage1/ZComponent/ZAccumulator2 ==
  op : Inport
  x : Inport  Port=2
  y : Inport  Port=3
  Sum1 : Sum  Inputs=|++  OutDataTypeStr=Inherit: Same as first input
  Sum2 : Sum  Inputs=|+-  OutDataTypeStr=Inherit: Same as first input
  Switch : Switch  Criteria=u2 ~= 0  OutDataTypeStr=Inherit: Inherit via back propagation
  Out1 : Outport
  wires:
  Switch/1 -> Out1/1
  Sum1/1 -> Switch/1
  op/1 -> Switch/2
  Sum2/1 -> Switch/3
  x/1 -> Sum2/1, Sum1/1
  y/1 -> Sum2/2, Sum1/2

== system sdruFMMonoFPGA/FM Receiver/FM_Demod_FPGA/FM Demodulator/cordic_arctan/cordic_stage2/XComponent/ZAccumulator2 ==
  y : Inport
  op : Inport  Port=2
  x : Inport  Port=3
  Sum1 : Sum  Inputs=|++  OutDataTypeStr=Inherit: Same as first input
  Sum2 : Sum  Inputs=|+-  OutDataTypeStr=Inherit: Same as first input
  Switch : Switch  Criteria=u2 ~= 0
  Out1 : Outport
  wires:
  y/1 -> Sum2/2, Sum1/2
  x/1 -> Sum2/1, Sum1/1
  Sum2/1 -> Switch/3
  op/1 -> Switch/2
  Sum1/1 -> Switch/1
  Switch/1 -> Out1/1

== system sdruFMMonoFPGA/FM Receiver/FM_Demod_FPGA/FM Demodulator/cordic_arctan/cordic_stage2/YComponent/ZAccumulator2 ==
  x : Inport
  op : Inport  Port=2
  y : Inport  Port=3
  Sum1 : Sum  Inputs=|++  OutDataTypeStr=Inherit: Same as first input
  Sum2 : Sum  Inputs=|+-  OutDataTypeStr=Inherit: Same as first input
  Switch : Switch  Criteria=u2 ~= 0  InputSameDT=on
  Out1 : Outport
  wires:
  y/1 -> Sum2/1, Sum1/1
  Sum2/1 -> Switch/3
  op/1 -> Switch/2
  Sum1/1 -> Switch/1
  Switch/1 -> Out1/1
  x/1 -> Sum2/2, Sum1/2

== system sdruFMMonoFPGA/FM Receiver/FM_Demod_FPGA/FM Demodulator/cordic_arctan/cordic_stage2/ZComponent/ZAccumulator2 ==
  op : Inport
  x : Inport  Port=2
  y : Inport  Port=3
  Sum1 : Sum  Inputs=|++  OutDataTypeStr=Inherit: Same as first input
  Sum2 : Sum  Inputs=|+-  OutDataTypeStr=Inherit: Same as first input
  Switch : Switch  Criteria=u2 ~= 0  OutDataTypeStr=Inherit: Inherit via back propagation
  Out1 : Outport
  wires:
  y/1 -> Sum1/2, Sum2/2
  x/1 -> Sum1/1, Sum2/1
  Sum2/1 -> Switch/3
  op/1 -> Switch/2
  Sum1/1 -> Switch/1
  Switch/1 -> Out1/1

== system sdruFMMonoFPGA/FM Receiver/FM_Demod_FPGA/FM Demodulator/cordic_arctan/cordic_stage3/XComponent/ZAccumulator2 ==
  y : Inport
  op : Inport  Port=2
  x : Inport  Port=3
  Sum1 : Sum  Inputs=|++  OutDataTypeStr=Inherit: Same as first input
  Sum2 : Sum  Inputs=|+-  OutDataTypeStr=Inherit: Same as first input
  Switch : Switch  Criteria=u2 ~= 0
  Out1 : Outport
  wires:
  Switch/1 -> Out1/1
  Sum1/1 -> Switch/1
  op/1 -> Switch/2
  Sum2/1 -> Switch/3
  x/1 -> Sum1/1, Sum2/1
  y/1 -> Sum1/2, Sum2/2

== system sdruFMMonoFPGA/FM Receiver/FM_Demod_FPGA/FM Demodulator/cordic_arctan/cordic_stage3/YComponent/ZAccumulator2 ==
  x : Inport
  op : Inport  Port=2
  y : Inport  Port=3
  Sum1 : Sum  Inputs=|++  OutDataTypeStr=Inherit: Same as first input
  Sum2 : Sum  Inputs=|+-  OutDataTypeStr=Inherit: Same as first input
  Switch : Switch  Criteria=u2 ~= 0  InputSameDT=on
  Out1 : Outport
  wires:
  x/1 -> Sum1/2, Sum2/2
  Switch/1 -> Out1/1
  Sum1/1 -> Switch/1
  op/1 -> Switch/2
  Sum2/1 -> Switch/3
  y/1 -> Sum1/1, Sum2/1

== system sdruFMMonoFPGA/FM Receiver/FM_Demod_FPGA/FM Demodulator/cordic_arctan/cordic_stage3/ZComponent/ZAccumulator2 ==
  op : Inport
  x : Inport  Port=2
  y : Inport  Port=3
  Sum1 : Sum  Inputs=|++  OutDataTypeStr=Inherit: Same as first input
  Sum2 : Sum  Inputs=|+-  OutDataTypeStr=Inherit: Same as first input
  Switch : Switch  Criteria=u2 ~= 0  OutDataTypeStr=Inherit: Inherit via back propagation
  Out1 : Outport
  wires:
  Switch/1 -> Out1/1
  Sum1/1 -> Switch/1
  op/1 -> Switch/2
  Sum2/1 -> Switch/3
  x/1 -> Sum2/1, Sum1/1
  y/1 -> Sum2/2, Sum1/2

== system sdruFMMonoFPGA/FM Receiver/FM_Demod_FPGA/FM Demodulator/cordic_arctan/cordic_stage4/XComponent/ZAccumulator2 ==
  y : Inport
  op : Inport  Port=2
  x : Inport  Port=3
  Sum1 : Sum  Inputs=|++  OutDataTypeStr=Inherit: Same as first input
  Sum2 : Sum  Inputs=|+-  OutDataTypeStr=Inherit: Same as first input
  Switch : Switch  Criteria=u2 ~= 0
  Out1 : Outport
  wires:
  y/1 -> Sum2/2, Sum1/2
  x/1 -> Sum2/1, Sum1/1
  Sum2/1 -> Switch/3
  op/1 -> Switch/2
  Sum1/1 -> Switch/1
  Switch/1 -> Out1/1

== system sdruFMMonoFPGA/FM Receiver/FM_Demod_FPGA/FM Demodulator/cordic_arctan/cordic_stage4/YComponent/ZAccumulator2 ==
  x : Inport
  op : Inport  Port=2
  y : Inport  Port=3
  Sum1 : Sum  Inputs=|++  OutDataTypeStr=Inherit: Same as first input
  Sum2 : Sum  Inputs=|+-  OutDataTypeStr=Inherit: Same as first input
  Switch : Switch  Criteria=u2 ~= 0  InputSameDT=on
  Out1 : Outport
  wires:
  y/1 -> Sum2/1, Sum1/1
  Sum2/1 -> Switch/3
  op/1 -> Switch/2
  Sum1/1 -> Switch/1
  Switch/1 -> Out1/1
  x/1 -> Sum2/2, Sum1/2

== system sdruFMMonoFPGA/FM Receiver/FM_Demod_FPGA/FM Demodulator/cordic_arctan/cordic_stage4/ZComponent/ZAccumulator2 ==
  op : Inport
  x : Inport  Port=2
  y : Inport  Port=3
  Sum1 : Sum  Inputs=|++  OutDataTypeStr=Inherit: Same as first input
  Sum2 : Sum  Inputs=|+-  OutDataTypeStr=Inherit: Same as first input
  Switch : Switch  Criteria=u2 ~= 0  OutDataTypeStr=Inherit: Inherit via back propagation
  Out1 : Outport
  wires:
  y/1 -> Sum1/2, Sum2/2
  x/1 -> Sum1/1, Sum2/1
  Sum2/1 -> Switch/3
  op/1 -> Switch/2
  Sum1/1 -> Switch/1
  Switch/1 -> Out1/1

== system sdruFMMonoFPGA/FM Receiver/FM_Demod_FPGA/FM Demodulator/cordic_arctan/cordic_stage5/XComponent/ZAccumulator2 ==
  y : Inport
  op : Inport  Port=2
  x : Inport  Port=3
  Sum1 : Sum  Inputs=|++  OutDataTypeStr=Inherit: Same as first input
  Sum2 : Sum  Inputs=|+-  OutDataTypeStr=Inherit: Same as first input
  Switch : Switch  Criteria=u2 ~= 0
  Out1 : Outport
  wires:
  Switch/1 -> Out1/1
  Sum1/1 -> Switch/1
  op/1 -> Switch/2
  Sum2/1 -> Switch/3
  x/1 -> Sum1/1, Sum2/1
  y/1 -> Sum1/2, Sum2/2

== system sdruFMMonoFPGA/FM Receiver/FM_Demod_FPGA/FM Demodulator/cordic_arctan/cordic_stage5/YComponent/ZAccumulator2 ==
  x : Inport
  op : Inport  Port=2
  y : Inport  Port=3
  Sum1 : Sum  Inputs=|++  OutDataTypeStr=Inherit: Same as first input
  Sum2 : Sum  Inputs=|+-  OutDataTypeStr=Inherit: Same as first input
  Switch : Switch  Criteria=u2 ~= 0  InputSameDT=on
  Out1 : Outport
  wires:
  x/1 -> Sum1/2, Sum2/2
  Switch/1 -> Out1/1
  Sum1/1 -> Switch/1
  op/1 -> Switch/2
  Sum2/1 -> Switch/3
  y/1 -> Sum1/1, Sum2/1

== system sdruFMMonoFPGA/FM Receiver/FM_Demod_FPGA/FM Demodulator/cordic_arctan/cordic_stage5/ZComponent/ZAccumulator2 ==
  op : Inport
  x : Inport  Port=2
  y : Inport  Port=3
  Sum1 : Sum  Inputs=|++  OutDataTypeStr=Inherit: Same as first input
  Sum2 : Sum  Inputs=|+-  OutDataTypeStr=Inherit: Same as first input
  Switch : Switch  Criteria=u2 ~= 0  OutDataTypeStr=Inherit: Inherit via back propagation
  Out1 : Outport
  wires:
  Switch/1 -> Out1/1
  Sum1/1 -> Switch/1
  op/1 -> Switch/2
  Sum2/1 -> Switch/3
  x/1 -> Sum2/1, Sum1/1
  y/1 -> Sum2/2, Sum1/2

== system sdruFMMonoFPGA/FM Receiver/FM_Demod_FPGA/FM Demodulator/cordic_arctan/cordic_stage6/XComponent/ZAccumulator2 ==
  y : Inport
  op : Inport  Port=2
  x : Inport  Port=3
  Sum1 : Sum  Inputs=|++  OutDataTypeStr=Inherit: Same as first input
  Sum2 : Sum  Inputs=|+-  OutDataTypeStr=Inherit: Same as first input
  Switch : Switch  Criteria=u2 ~= 0
  Out1 : Outport
  wires:
  y/1 -> Sum2/2, Sum1/2
  x/1 -> Sum2/1, Sum1/1
  Sum2/1 -> Switch/3
  op/1 -> Switch/2
  Sum1/1 -> Switch/1
  Switch/1 -> Out1/1

== system sdruFMMonoFPGA/FM Receiver/FM_Demod_FPGA/FM Demodulator/cordic_arctan/cordic_stage6/YComponent/ZAccumulator2 ==
  x : Inport
  op : Inport  Port=2
  y : Inport  Port=3
  Sum1 : Sum  Inputs=|++  OutDataTypeStr=Inherit: Same as first input
  Sum2 : Sum  Inputs=|+-  OutDataTypeStr=Inherit: Same as first input
  Switch : Switch  Criteria=u2 ~= 0  InputSameDT=on
  Out1 : Outport
  wires:
  y/1 -> Sum2/1, Sum1/1
  Sum2/1 -> Switch/3
  op/1 -> Switch/2
  Sum1/1 -> Switch/1
  Switch/1 -> Out1/1
  x/1 -> Sum2/2, Sum1/2

== system sdruFMMonoFPGA/FM Receiver/FM_Demod_FPGA/FM Demodulator/cordic_arctan/cordic_stage6/ZComponent/ZAccumulator2 ==
  op : Inport
  x : Inport  Port=2
  y : Inport  Port=3
  Sum1 : Sum  Inputs=|++  OutDataTypeStr=Inherit: Same as first input
  Sum2 : Sum  Inputs=|+-  OutDataTypeStr=Inherit: Same as first input
  Switch : Switch  Criteria=u2 ~= 0  OutDataTypeStr=Inherit: Inherit via back propagation
  Out1 : Outport
  wires:
  y/1 -> Sum1/2, Sum2/2
  x/1 -> Sum1/1, Sum2/1
  Sum2/1 -> Switch/3
  op/1 -> Switch/2
  Sum1/1 -> Switch/1
  Switch/1 -> Out1/1

== system sdruFMMonoFPGA/FM Receiver/FM_Demod_FPGA/FM Demodulator/cordic_arctan/cordic_stage7/XComponent/ZAccumulator2 ==
  y : Inport
  op : Inport  Port=2
  x : Inport  Port=3
  Sum1 : Sum  Inputs=|++  OutDataTypeStr=Inherit: Same as first input
  Sum2 : Sum  Inputs=|+-  OutDataTypeStr=Inherit: Same as first input
  Switch : Switch  Criteria=u2 ~= 0
  Out1 : Outport
  wires:
  Switch/1 -> Out1/1
  Sum1/1 -> Switch/1
  op/1 -> Switch/2
  Sum2/1 -> Switch/3
  x/1 -> Sum1/1, Sum2/1
  y/1 -> Sum1/2, Sum2/2

== system sdruFMMonoFPGA/FM Receiver/FM_Demod_FPGA/FM Demodulator/cordic_arctan/cordic_stage7/YComponent/ZAccumulator2 ==
  x : Inport
  op : Inport  Port=2
  y : Inport  Port=3
  Sum1 : Sum  Inputs=|++  OutDataTypeStr=Inherit: Same as first input
  Sum2 : Sum  Inputs=|+-  OutDataTypeStr=Inherit: Same as first input
  Switch : Switch  Criteria=u2 ~= 0  InputSameDT=on
  Out1 : Outport
  wires:
  x/1 -> Sum1/2, Sum2/2
  Switch/1 -> Out1/1
  Sum1/1 -> Switch/1
  op/1 -> Switch/2
  Sum2/1 -> Switch/3
  y/1 -> Sum1/1, Sum2/1

== system sdruFMMonoFPGA/FM Receiver/FM_Demod_FPGA/FM Demodulator/cordic_arctan/cordic_stage7/ZComponent/ZAccumulator2 ==
  op : Inport
  x : Inport  Port=2
  y : Inport  Port=3
  Sum1 : Sum  Inputs=|++  OutDataTypeStr=Inherit: Same as first input
  Sum2 : Sum  Inputs=|+-  OutDataTypeStr=Inherit: Same as first input
  Switch : Switch  Criteria=u2 ~= 0  OutDataTypeStr=Inherit: Inherit via back propagation
  Out1 : Outport
  wires:
  Switch/1 -> Out1/1
  Sum1/1 -> Switch/1
  op/1 -> Switch/2
  Sum2/1 -> Switch/3
  x/1 -> Sum2/1, Sum1/1
  y/1 -> Sum2/2, Sum1/2

== system sdruFMMonoFPGA/FM Receiver/FM_Demod_FPGA/FM Demodulator/cordic_arctan/cordic_stage8/XComponent/ZAccumulator2 ==
  y : Inport
  op : Inport  Port=2
  x : Inport  Port=3
  Sum1 : Sum  Inputs=|++  OutDataTypeStr=Inherit: Same as first input
  Sum2 : Sum  Inputs=|+-  OutDataTypeStr=Inherit: Same as first input
  Switch : Switch  Criteria=u2 ~= 0
  Out1 : Outport
  wires:
  y/1 -> Sum2/2, Sum1/2
  x/1 -> Sum2/1, Sum1/1
  Sum2/1 -> Switch/3
  op/1 -> Switch/2
  Sum1/1 -> Switch/1
  Switch/1 -> Out1/1

== system sdruFMMonoFPGA/FM Receiver/FM_Demod_FPGA/FM Demodulator/cordic_arctan/cordic_stage8/YComponent/ZAccumulator2 ==
  x : Inport
  op : Inport  Port=2
  y : Inport  Port=3
  Sum1 : Sum  Inputs=|++  OutDataTypeStr=Inherit: Same as first input
  Sum2 : Sum  Inputs=|+-  OutDataTypeStr=Inherit: Same as first input
  Switch : Switch  Criteria=u2 ~= 0  InputSameDT=on
  Out1 : Outport
  wires:
  y/1 -> Sum2/1, Sum1/1
  Sum2/1 -> Switch/3
  op/1 -> Switch/2
  Sum1/1 -> Switch/1
  Switch/1 -> Out1/1
  x/1 -> Sum2/2, Sum1/2

== system sdruFMMonoFPGA/FM Receiver/FM_Demod_FPGA/FM Demodulator/cordic_arctan/cordic_stage8/ZComponent/ZAccumulator2 ==
  op : Inport
  x : Inport  Port=2
  y : Inport  Port=3
  Sum1 : Sum  Inputs=|++  OutDataTypeStr=Inherit: Same as first input
  Sum2 : Sum  Inputs=|+-  OutDataTypeStr=Inherit: Same as first input
  Switch : Switch  Criteria=u2 ~= 0  OutDataTypeStr=Inherit: Inherit via back propagation
  Out1 : Outport
  wires:
  y/1 -> Sum1/2, Sum2/2
  x/1 -> Sum1/1, Sum2/1
  Sum2/1 -> Switch/3
  op/1 -> Switch/2
  Sum1/1 -> Switch/1
  Switch/1 -> Out1/1
